simulink library "xrbsComm_r3"  (Simulink 5.1)
libraries: xbsIndex_r3 x775, xrbsComm_r3 x1
(part 6 of 6)

== system xrbsComm_r3/White Gaussian  Noise Generator/Box-Muller4/g2/lfsr_47_5/x12/ASR ==
  din : Inport
  Addressable Shift Register : xbsIndex_r3/Addressable Shift Register  infer_latency=off  depth=asr_length  initVector=init  explicit_period=off  period=-1  accept_only_valid=off  en=off  dbl_ovrd=off  gen_core=on  use_rpm=off
      settings: xl_area=[0, 0, 0, 0, 0, 0, 0]
  Constant1 : xbsIndex_r3/Constant  const=asr_length-1  arith_type=Unsigned  n_bits=size(dec2bin(asr_length-1),2)  bin_pt=0  explicit_period=off  period=1  dbl_ovrd=off
  dout : Outport
  wires:
  Constant1/1 -> Addressable Shift Register/2
  Addressable Shift Register/1 -> dout/1
  din/1 -> Addressable Shift Register/1

== system xrbsComm_r3/White Gaussian  Noise Generator/Box-Muller4/g2/lfsr_47_5/x13/ASR ==
  din : Inport
  Addressable Shift Register : xbsIndex_r3/Addressable Shift Register  infer_latency=off  depth=asr_length  initVector=init  explicit_period=off  period=-1  accept_only_valid=off  en=off  dbl_ovrd=off  gen_core=on  use_rpm=off
      settings: xl_area=[0, 0, 0, 0, 0, 0, 0]
  Constant1 : xbsIndex_r3/Constant  const=asr_length-1  arith_type=Unsigned  n_bits=size(dec2bin(asr_length-1),2)  bin_pt=0  explicit_period=off  period=1  dbl_ovrd=off
  dout : Outport
  wires:
  Constant1/1 -> Addressable Shift Register/2
  Addressable Shift Register/1 -> dout/1
  din/1 -> Addressable Shift Register/1

== system xrbsComm_r3/White Gaussian  Noise Generator/Box-Muller4/g2/lfsr_47_5/x14/ASR ==
  din : Inport
  Addressable Shift Register : xbsIndex_r3/Addressable Shift Register  infer_latency=off  depth=asr_length  initVector=init  explicit_period=off  period=-1  accept_only_valid=off  en=off  dbl_ovrd=off  gen_core=on  use_rpm=off
      settings: xl_area=[0, 0, 0, 0, 0, 0, 0]
  Constant1 : xbsIndex_r3/Constant  const=asr_length-1  arith_type=Unsigned  n_bits=size(dec2bin(asr_length-1),2)  bin_pt=0  explicit_period=off  period=1  dbl_ovrd=off
  dout : Outport
  wires:
  Constant1/1 -> Addressable Shift Register/2
  Addressable Shift Register/1 -> dout/1
  din/1 -> Addressable Shift Register/1

== system xrbsComm_r3/White Gaussian  Noise Generator/Box-Muller4/g2/lfsr_47_5/x15/ASR ==
  din : Inport
  Addressable Shift Register : xbsIndex_r3/Addressable Shift Register  infer_latency=off  depth=asr_length  initVector=init  explicit_period=off  period=-1  accept_only_valid=off  en=off  dbl_ovrd=off  gen_core=on  use_rpm=off
      settings: xl_area=[0, 0, 0, 0, 0, 0, 0]
  Constant1 : xbsIndex_r3/Constant  const=asr_length-1  arith_type=Unsigned  n_bits=size(dec2bin(asr_length-1),2)  bin_pt=0  explicit_period=off  period=1  dbl_ovrd=off
  dout : Outport
  wires:
  Constant1/1 -> Addressable Shift Register/2
  Addressable Shift Register/1 -> dout/1
  din/1 -> Addressable Shift Register/1

== system xrbsComm_r3/White Gaussian  Noise Generator/Box-Muller4/g2/lfsr_47_5/x16/ASR ==
  din : Inport
  Addressable Shift Register : xbsIndex_r3/Addressable Shift Register  infer_latency=off  depth=asr_length  initVector=init  explicit_period=off  period=-1  accept_only_valid=off  en=off  dbl_ovrd=off  gen_core=on  use_rpm=off
      settings: xl_area=[0, 0, 0, 0, 0, 0, 0]
  Constant1 : xbsIndex_r3/Constant  const=asr_length-1  arith_type=Unsigned  n_bits=size(dec2bin(asr_length-1),2)  bin_pt=0  explicit_period=off  period=1  dbl_ovrd=off
  dout : Outport
  wires:
  Constant1/1 -> Addressable Shift Register/2
  Addressable Shift Register/1 -> dout/1
  din/1 -> Addressable Shift Register/1

== system xrbsComm_r3/White Gaussian  Noise Generator/Box-Muller4/g2/lfsr_47_5/x9/ASR ==
  din : Inport
  Addressable Shift Register : xbsIndex_r3/Addressable Shift Register  infer_latency=off  depth=asr_length  initVector=init  explicit_period=off  period=-1  accept_only_valid=off  en=off  dbl_ovrd=off  gen_core=on  use_rpm=off
      settings: xl_area=[0, 0, 0, 0, 0, 0, 0]
  Constant1 : xbsIndex_r3/Constant  const=asr_length-1  arith_type=Unsigned  n_bits=size(dec2bin(asr_length-1),2)  bin_pt=0  explicit_period=off  period=1  dbl_ovrd=off
  dout : Outport
  wires:
  Constant1/1 -> Addressable Shift Register/2
  Addressable Shift Register/1 -> dout/1
  din/1 -> Addressable Shift Register/1
